simulink model "sampleModel2048"  (R2023a)
settings: Solver=VariableStepAuto  StartTime=0.0  StopTime=10.0  RelTol=1e-3
libraries: hdlsllib x4, simulink x3
settings Model: Creator=user1  LastModifiedBy=user1

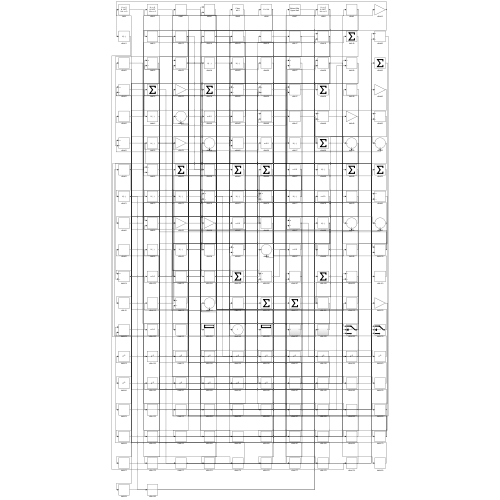
[thumbnail: Simulink's stored preview of the top-level diagram]
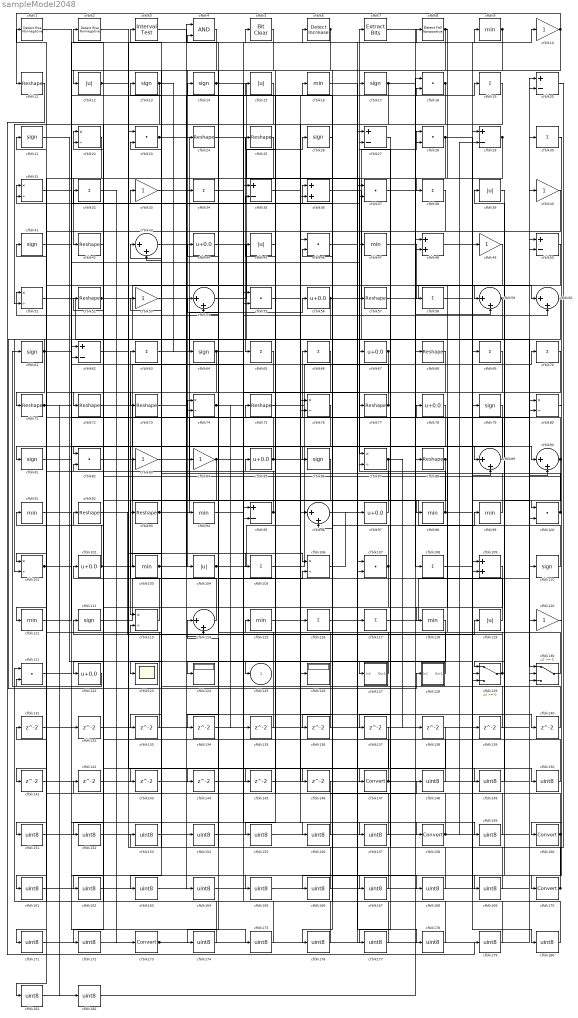
== system sampleModel2048 ==
  cfblk1 : hdlsllib/Logic and Bit Operations/Detect Rise Nonnegative  vinit=0  OutDataTypeStr=boolean
  cfblk{10,33,40,49,53,83..84,120} (8 alike) : Gain
  cfblk{18,23,28,37,46,55,82,100,107,121} (10 alike) : DotProduct  OutDataTypeStr=Inherit: Inherit via internal rule
  cfblk{22,31,51,74,76,80,87,101,106,113} (10 alike) : Product  Inputs=*/  RndMeth=Zero  SaturateOnIntegerOverflow=on
  cfblk{44,56,67,78,85,97,102,122} (8 alike) : Bias  Bias=0.0  SaturateOnIntegerOverflow=off
  cfblk{9,16,47,91,94,98..99,103,111,115,118} (11 alike) : MinMax
  cfblk{12,15,39,45,104,119} (6 alike) : Abs  SaturateOnIntegerOverflow=off
  cfblk{19,30,32,34,38,58,63,65..66,69..70,105,108,116..117} (15 alike) : Sum  Inputs=+
  cfblk109 : Sum
  cfblk{11,24..25,42,52,57,68,71..73,75,77,88,92..93} (15 alike) : Reshape
  cfblk{13..14,17,21,26,41,61,64,79,81,86,110,112} (13 alike) : Signum
  cfblk{43,54,59..60,89..90,96,114} (8 alike) : Sum  Inputs=|++
  cfblk123 : Scope
  cfblk124 : Display
  cfblk126 : Display
  cfblk127 : Subsystem
      settings: LibrarySourceBlock=|
      | hdlsllib/Ports &
      | Subsystems/Subsystem
  cfblk128 : Subsystem
      settings: LibrarySourceBlock=|
      | hdlsllib/Ports &
      | Subsystems/Subsystem
  cfblk129 : Switch  SaturateOnIntegerOverflow=off  InputSameDT=off
  cfblk130 : Switch  SaturateOnIntegerOverflow=off  InputSameDT=off
  cfblk{131..146} (16 alike) : Delay  SampleTime=1
  cfblk{147,158,160,170,173} (5 alike) : DataTypeConversion  SaturateOnIntegerOverflow=off  RndMeth=Floor
  cfblk{148..157,159,161..169,171..172,174..182} (31 alike) : DataTypeConversion  OutDataTypeStr=uint8  SaturateOnIntegerOverflow=off  RndMeth=Floor
  cfblk2 : hdlsllib/Logic and Bit Operations/Detect Rise Nonnegative  vinit=0  OutDataTypeStr=boolean
  cfblk{20,27,29,35,50,62,95} (7 alike) : Sum  Inputs=+-
  cfblk3 : hdlsllib/Logic and Bit Operations/Interval Test  IntervalClosedRight=on  uplimit=0.5  IntervalClosedLeft=on  lowlimit=-0.5  OutDataTypeStr=boolean
  cfblk36 : Sum
  cfblk4 : Logic  AllPortsSameDT=off  OutDataTypeStr=boolean
  cfblk48 : Sum
  cfblk5 : simulink/Logic and Bit Operations/Bit Clear  iBit=0
      settings: LibrarySourceBlock=|
      | hdlsllib/Logic and Bit
      | Operations/Bit Clear
  cfblk6 : simulink/Logic and Bit Operations/Detect Increase  vinit=0.0  OutDataTypeStr=boolean
      settings: LibrarySourceBlock=|
      | hdlsllib/Logic and Bit
      | Operations/Detect
      | Increase
  cfblk7 : simulink/Logic and Bit Operations/Extract Bits  bitsToExtract=Upper half  numBits=8  bitIdxRange=[0 7]  outScalingMode=Preserve fixed-point scaling
      settings: LibrarySourceBlock=|
      | hdlsllib/Logic and Bit
      | Operations/Extract Bits
  cfblk8 : hdlsllib/Logic and Bit Operations/Detect Fall Nonpositive  vinit=0  OutDataTypeStr=boolean
  cfblk125 : Outport  VectorParamsAs1DForOutWhenUnconnected=off
  wires:
  cfblk98/1 -> cfblk7/1, cfblk10/1
  cfblk22/1 -> cfblk42/1
  cfblk89/1 -> cfblk66/1
  cfblk32/1 -> cfblk173/1
  cfblk23/1 -> cfblk99/1, cfblk114/2
  cfblk21/1 -> cfblk127/1(In1)
  cfblk88/1 -> cfblk136/1, cfblk137/1
  cfblk113/1 -> cfblk63/1
  cfblk15/1 -> cfblk72/1
  cfblk42/1 -> cfblk82/1
  cfblk72/1 -> cfblk90/1
  cfblk2/1 -> cfblk147/1
  cfblk18/1 -> cfblk104/1, cfblk76/2
  cfblk106/1 -> cfblk97/1
  cfblk24/1 -> cfblk65/1
  cfblk81/1 -> cfblk74/1
  cfblk44/1 -> cfblk110/1
  cfblk92/1 -> cfblk119/1
  cfblk29/1 -> cfblk141/1, cfblk174/1
  cfblk6/1 -> cfblk123/1, cfblk73/1
  cfblk5/1 -> cfblk24/1
  cfblk57/1 -> cfblk59/1
  cfblk58/1 -> cfblk79/1
  cfblk105/1 -> cfblk70/1
  cfblk74/1 -> cfblk129/2, cfblk135/1
  cfblk76/1 -> cfblk81/1
  cfblk116/1 -> cfblk117/1
  cfblk67/1 -> cfblk122/1, cfblk145/1
  cfblk129/1 -> cfblk112/1, cfblk51/1
  cfblk56/1 -> cfblk28/1, cfblk101/2
  cfblk51/1 -> cfblk108/1
  cfblk54/1 -> cfblk26/1
  cfblk102/1 -> cfblk35/1, cfblk22/1, cfblk31/2, cfblk37/2
  cfblk100/1 -> cfblk43/1, cfblk22/2
  cfblk75/1 -> cfblk29/1
  cfblk96/1 -> cfblk9/1
  cfblk94/1 -> cfblk36/1
  cfblk17/1 -> cfblk125/1, cfblk60/1
  cfblk120/1 -> cfblk160/1
  cfblk63/1 -> cfblk56/1
  cfblk117/1 -> cfblk50/1
  cfblk93/1 -> cfblk49/1, cfblk140/1
  cfblk122/1 -> cfblk61/1
  cfblk34/1 -> cfblk8/1
  cfblk80/1 -> cfblk170/1
  cfblk35/1 -> cfblk126/1
  cfblk14/1 -> cfblk87/1, cfblk129/3
  cfblk62/1 -> cfblk5/1
  cfblk103/1 -> cfblk17/1, cfblk75/1
  cfblk45/1 -> cfblk15/1
  cfblk68/1 -> cfblk124/1
  cfblk99/1 -> cfblk33/1
  cfblk26/1 -> cfblk96/2
  cfblk61/1 -> cfblk128/1(In1), cfblk47/1, cfblk71/1
  cfblk128/1(Out1) -> cfblk4/2
  cfblk30/1 -> cfblk100/1
  cfblk77/1 -> cfblk45/1, cfblk52/1
  cfblk12/1 -> cfblk106/1, cfblk105/1
  cfblk112/1 -> cfblk106/2
  cfblk114/1 -> cfblk92/1
  cfblk70/1 -> cfblk118/1
  cfblk97/1 -> cfblk87/2
  cfblk101/1 -> cfblk19/1, cfblk74/2
  cfblk52/1 -> cfblk90/2, cfblk55/2
  cfblk71/1 -> cfblk168/1, cfblk182/1
  cfblk33/1 -> cfblk67/1
  cfblk8/1 -> cfblk38/1, cfblk166/1
  cfblk79/1 -> cfblk111/1
  cfblk85/1 -> cfblk21/1, cfblk30/1
  cfblk10/1 -> cfblk11/1, cfblk155/1
  cfblk65/1 -> cfblk95/2
  cfblk110/1 -> cfblk14/1
  cfblk84/1 -> cfblk113/1, cfblk60/2
  cfblk95/1 -> cfblk25/1, cfblk41/1
  cfblk119/1 -> cfblk44/1
  cfblk9/1 -> cfblk84/1, cfblk12/1
  cfblk19/1 -> cfblk34/1
  cfblk107/1 -> cfblk31/1, cfblk133/1
  cfblk87/1 -> cfblk138/1, cfblk152/1
  cfblk127/1(Out1) -> cfblk54/1
  cfblk59/1 -> cfblk134/1, cfblk163/1
  cfblk130/1 -> cfblk78/1
  cfblk7/1 -> cfblk68/1
  cfblk111/1 -> cfblk6/1
  cfblk50/1 -> cfblk98/1
  cfblk25/1 -> cfblk54/2
  cfblk47/1 -> cfblk58/1
  cfblk4/1 -> cfblk62/2
  cfblk41/1 -> cfblk35/2
  cfblk28/1 -> cfblk101/1, cfblk86/1, cfblk100/2
  cfblk13/1 -> cfblk93/1, cfblk64/1, cfblk51/2
  cfblk86/1 -> cfblk103/1
  cfblk36/1 -> cfblk130/1
  cfblk55/1 -> cfblk18/2
  cfblk64/1 -> cfblk77/1, cfblk83/1
  cfblk115/1 -> cfblk158/1
  cfblk82/1 -> cfblk116/1
  cfblk37/1 -> cfblk59/2
  cfblk104/1 -> cfblk76/1, cfblk157/1
  cfblk90/1 -> cfblk43/2, cfblk129/1
  cfblk1/1 -> cfblk89/1
  cfblk38/1 -> cfblk94/1
  cfblk131/1 -> cfblk46/1
  cfblk31/1 -> cfblk132/1
  cfblk132/1 -> cfblk50/2
  cfblk133/1 -> cfblk1/1
  cfblk134/1 -> cfblk130/2
  cfblk135/1 -> cfblk4/1
  cfblk136/1 -> cfblk62/1
  cfblk108/1 -> cfblk139/1
  cfblk139/1 -> cfblk95/1
  cfblk140/1 -> cfblk23/2
  cfblk141/1 -> cfblk130/3
  cfblk142/1 -> cfblk36/2
  cfblk60/1 -> cfblk143/1
  cfblk143/1 -> cfblk28/2
  cfblk118/1 -> cfblk144/1
  cfblk144/1 -> cfblk96/1
  cfblk145/1 -> cfblk89/2
  cfblk69/1 -> cfblk146/1
  cfblk147/1 -> cfblk113/2, cfblk69/1, cfblk85/1
  cfblk146/1 -> cfblk148/1
  cfblk148/1 -> cfblk2/1
  cfblk3/1 -> cfblk149/1
  cfblk149/1 -> cfblk39/1
  cfblk46/1 -> cfblk150/1
  cfblk150/1 -> cfblk3/1
  cfblk40/1 -> cfblk151/1
  cfblk151/1 -> cfblk88/1
  cfblk152/1 -> cfblk40/1
  cfblk20/1 -> cfblk153/1
  cfblk153/1 -> cfblk37/1
  cfblk73/1 -> cfblk154/1
  cfblk154/1 -> cfblk20/1
  cfblk155/1 -> cfblk20/2
  cfblk91/1 -> cfblk156/1
  cfblk156/1 -> cfblk102/1
  cfblk157/1 -> cfblk91/1
  cfblk158/1 -> cfblk142/1, cfblk29/2
  cfblk83/1 -> cfblk159/1
  cfblk159/1 -> cfblk115/1
  cfblk160/1 -> cfblk82/2, cfblk176/1
  cfblk49/1 -> cfblk161/1
  cfblk161/1 -> cfblk120/1
  cfblk109/1 -> cfblk162/1
  cfblk162/1 -> cfblk107/2
  cfblk163/1 -> cfblk109/1
  cfblk43/1 -> cfblk164/1
  cfblk164/1 -> cfblk109/2
  cfblk53/1 -> cfblk165/1
  cfblk165/1 -> cfblk107/1
  cfblk166/1 -> cfblk53/1
  cfblk27/1 -> cfblk167/1
  cfblk167/1 -> cfblk13/1
  cfblk168/1 -> cfblk27/1
  cfblk39/1 -> cfblk169/1
  cfblk169/1 -> cfblk27/2
  cfblk170/1 -> cfblk114/1, cfblk23/1
  cfblk66/1 -> cfblk171/1
  cfblk171/1 -> cfblk80/1
  cfblk137/1 -> cfblk172/1
  cfblk172/1 -> cfblk80/2
  cfblk173/1 -> cfblk57/1, cfblk18/1
  cfblk174/1 -> cfblk32/1
  cfblk121/1 -> cfblk175/1
  cfblk175/1 -> cfblk55/1
  cfblk176/1 -> cfblk121/1
  cfblk138/1 -> cfblk177/1
  cfblk177/1 -> cfblk121/2
  cfblk16/1 -> cfblk178/1
  cfblk178/1 -> cfblk131/1
  cfblk11/1 -> cfblk179/1
  cfblk179/1 -> cfblk16/1
  cfblk48/1 -> cfblk180/1
  cfblk180/1 -> cfblk46/2
  cfblk78/1 -> cfblk181/1
  cfblk181/1 -> cfblk48/1
  cfblk182/1 -> cfblk48/2

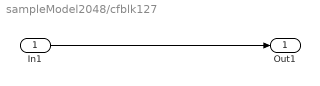
== system sampleModel2048/cfblk127 ==
  In1 : Inport
  Out1 : Outport
  wires:
  In1/1 -> Out1/1

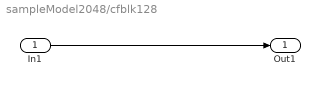
== system sampleModel2048/cfblk128 ==
  In1 : Inport
  Out1 : Outport
  wires:
  In1/1 -> Out1/1
